simulink model "Balloon"  (R2022a)
settings: Solver=FixedStepAuto  StartTime=0.0  StopTime=25  RelTol=1e-3
values from neighbouring files (symbols this model uses):
  alpha = T0/Tup    (= 0.509048214605)    [in.m]
  g = 9.8    [in.m]
  h0 = 100    [in.m]
  M = 100    [in.m]
  m = 200    [in.m]
  rho0 = 1.2    [in.m]
  V = 500    [in.m]
libraries: simulink x1, sldrtlib x1
settings Model: Creator=Daddy  LastModifiedBy=ilyas
settings SolverCC: ZeroCrossControl=DisableAll  ZeroCrossAlgorithm=Adaptive  AlgebraicLoopSolver=TrustRegion
settings DataIOCC: LimitDataPoints=on  SaveFormat=Array  ReturnWorkspaceOutputs=off
settings OptimizationCC: LifeSpan=inf
settings DebuggingCC: SolverPrmCheckMsg=warning  UnconnectedInputMsg=warning  UnconnectedOutputMsg=warning  UnconnectedLineMsg=warning  SFUnexpectedBacktrackingDiag=warning  SFNoUnconditionalDefaultTransitionDiag=warning  SFExecutionAtInitializationDiag=none  SFMachineParentedDataDiag=warning  ArithmeticOperatorsInVariantConditions=warning
settings HardwareCC: ProdBitPerPointer=32  ProdBitPerSizeT=32  ProdBitPerPtrDiffT=32  ProdLargestAtomicFloat=None  ProdIntDivRoundTo=Undefined  ProdEndianess=Unspecified  ProdWordSize=32  ProdHWDeviceType=32-bit Generic
settings ModelReferenceCC: PropagateSignalLabelsOutOfModel=off
settings SFSimCC: SimUseLocalCustomCode=off  CustomCodeUndefinedFunction=UseInterfaceOnly  SimTargetLang=C++
settings RTWCC: RTWUseLocalCustomCode=off
settings CodeAppCC: StateflowObjectComments=on
settings GRTTargetCC: TargetLangStandard=C89/C90 (ANSI)
settings ConfigComp: CovMetricSettings=dw  CovSaveCumulativeToWorkspaceVar=on  CovSaveSingleToWorkspaceVar=on  CovExternalEMLEnable=off  CovSFcnEnable=off

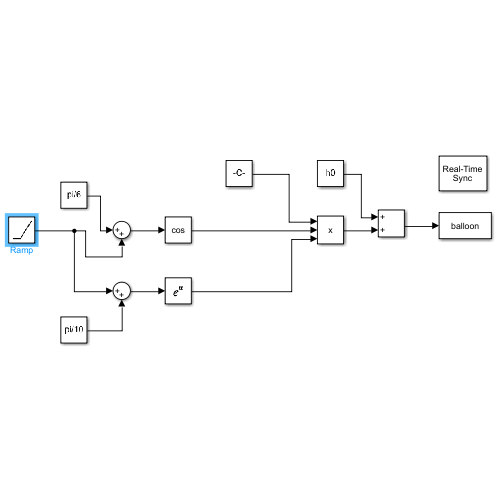
[thumbnail: Simulink's stored preview of the top-level diagram]
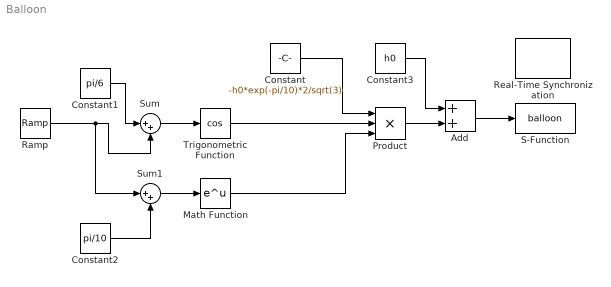
== system Balloon ==
  Add : Sum
  Constant : Constant  Value=-h0*exp(-pi/10)*2/sqrt(3)
  Constant1 : Constant  Value=pi/6
  Constant2 : Constant  Value=pi/10
  Constant3 : Constant  Value=h0
  Math Function : Math
  Product : Product  Inputs=3
  Ramp : simulink/Sources/Ramp  slope=g*(rho0*V*(1-alpha)-M-m)/(alpha*rho0 + M + m)  start=2.5  InitialOutput=0
  Real-Time Synchronization : sldrtlib/Real-Time Synchronization  SampleTime=0.1  MaxMissedTicks=10  ShowMissedTicks=off  YieldWhenWaiting=off
  S-Function : S-Function  FunctionName=balloon  Parameters=h0  SFunctionDeploymentMode=off  EnableBusSupport=off
  Sum : Sum  Inputs=|++
  Sum1 : Sum  Inputs=|++
  Trigonometric Function : Trigonometry  Operator=cos
  wires:
  Ramp/1 -> Sum1/1, Sum/2
  Constant/1 -> Product/1
  Trigonometric Function/1 -> Product/2
  Math Function/1 -> Product/3
  Product/1 -> Add/2
  Add/1 -> S-Function/1
  Constant1/1 -> Sum/1
  Sum/1 -> Trigonometric Function/1
  Sum1/1 -> Math Function/1
  Constant2/1 -> Sum1/2
  Constant3/1 -> Add/1
